simulink model "BatteryChargingSim"  (R2024b)
settings: Solver=VariableStepAuto  StartTime=0.0  StopTime=10  RelTol=1e-3

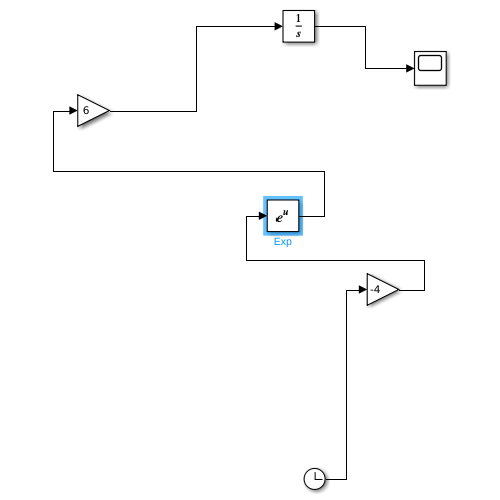
[thumbnail: Simulink's stored preview of the top-level diagram]
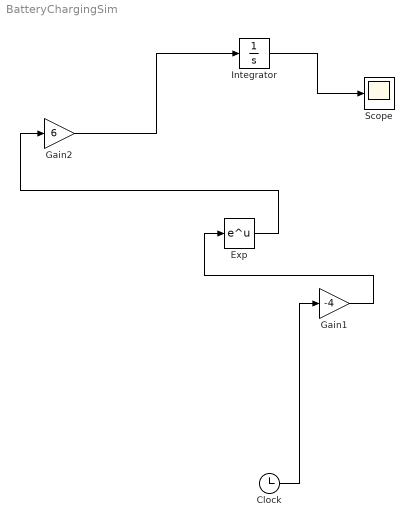
== system BatteryChargingSim ==
  Clock : Clock
  Exp : Math
  Gain1 : Gain  Gain=-4
  Gain2 : Gain  Gain=6
  Integrator : Integrator
  Scope : Scope
  wires:
  Clock/1 -> Gain1/1
  Gain1/1 -> Exp/1
  Exp/1 -> Gain2/1
  Gain2/1 -> Integrator/1
  Integrator/1 -> Scope/1
